simulink model "TP_7"  (R2023b)
settings: Solver=VariableStepAuto  StartTime=0.0  StopTime=0.1  RelTol=1e-3
libraries: spsIGBTDiodeLib x6, spsTriangleGeneratorLib x1, sps_lib x1
settings Model: Creator=sohayl  LastModifiedBy=sohayl

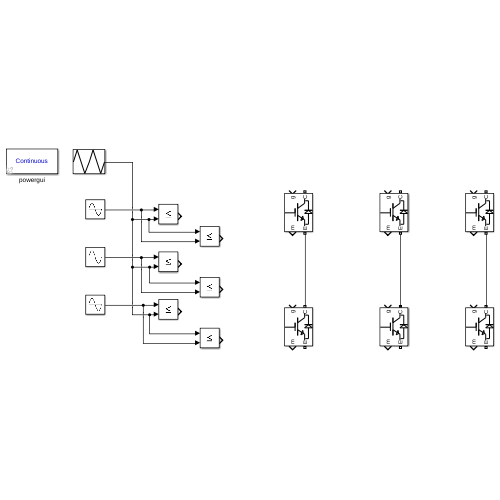
[thumbnail: Simulink's stored preview of the top-level diagram]
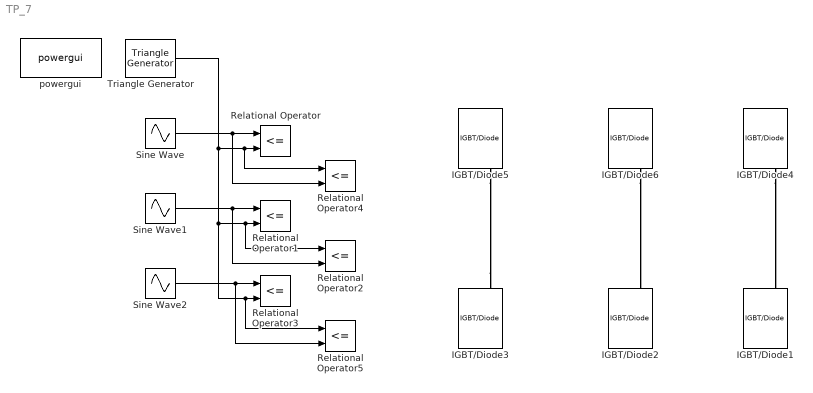
== system TP_7 ==
  IGBT/Diode{1..6} (6 alike) : spsIGBTDiodeLib/IGBT//Diode  Ron=1e-3  Rs=1e5  Cs=inf  Measurements=on
  Relational Operator{,1..5} (6 alike) : RelationalOperator  Operator=<=  OutDataTypeStr=boolean  RndMeth=Simplest  InputSameDT=off
  Sine Wave : Sin  Frequency=50  SampleTime=0
  Sine Wave1 : Sin  Frequency=50  Phase=2*pi/3  SampleTime=0
  Sine Wave2 : Sin  Frequency=50  Phase=4*pi/3  SampleTime=0
  Triangle Generator : spsTriangleGeneratorLib/Triangle Generator  Freq=60*6  Phase=90  Ts=0
  powergui : sps_lib/powergui  Priority=1  SimulationMode=Continuous  SampleTime=50e-6  frequency=60  Iterations=50  frequencyindice=60  Pbase=100e6  ErrMax=1e-4  UnitsV=kV  UnitsW=MW  buscounter=0  FunctionMessages=off  echomessages=off  EnableUseOfTLC=off  CurrentSourceSwitches=off  DisableSnubberDevices=off  DisableRonSwitches=off  DisableVfSwitches=off  DisplayEquations=off  AutomaticDiscreteSolvers=off  SolverType=Tustin/Backward Euler (TBE)  Interpol=off  ExternalGateDelay=off  methode=off  Ts=100  x0status=blocks  SPID=on  SwTol=0  HookPort=off  NonlinearTolerance=1e-4  nMaxIteration=100  ContinueOnMaxIteration=off  RestoreLinks=warning  ResistiveCurrentMeasurement=off  Frange=[0:2:500]  Ylog=off  Xlog=on  ShowGrid=off  save=off  variable=ZData  structure=0  ZoomFFT=off  StartTime=0.0  cycles=1  DisplayStyle=1  fundamental=60  FreqAxis=off  MaxFrequency=1000  frequencyindicesteady=1  RmsSteady=1  display=off
  wires:
  Sine Wave2/1 -> Relational Operator5/2, Relational Operator3/1
  Sine Wave1/1 -> Relational Operator2/2, Relational Operator1/1
  Sine Wave/1 -> Relational Operator4/2, Relational Operator/1
  Triangle Generator/1 -> Relational Operator5/1, Relational Operator3/2, Relational Operator2/1, Relational Operator1/2, Relational Operator4/1, Relational Operator/2
  connections:
  IGBT/Diode5/RConn1 -- IGBT/Diode3/LConn1
  IGBT/Diode6/RConn1 -- IGBT/Diode2/LConn1
  IGBT/Diode4/RConn1 -- IGBT/Diode1/LConn1
